simulink model "Feedback_linearization_3body_2body"  (R2019a)
settings: Solver=FixedStepAuto  StartTime=0.0  StopTime=5  FixedStep=0.001  RelTol=1e-7
libraries: simulink x1
settings Model: Creator=tommaso  LastModifiedBy=tommaso

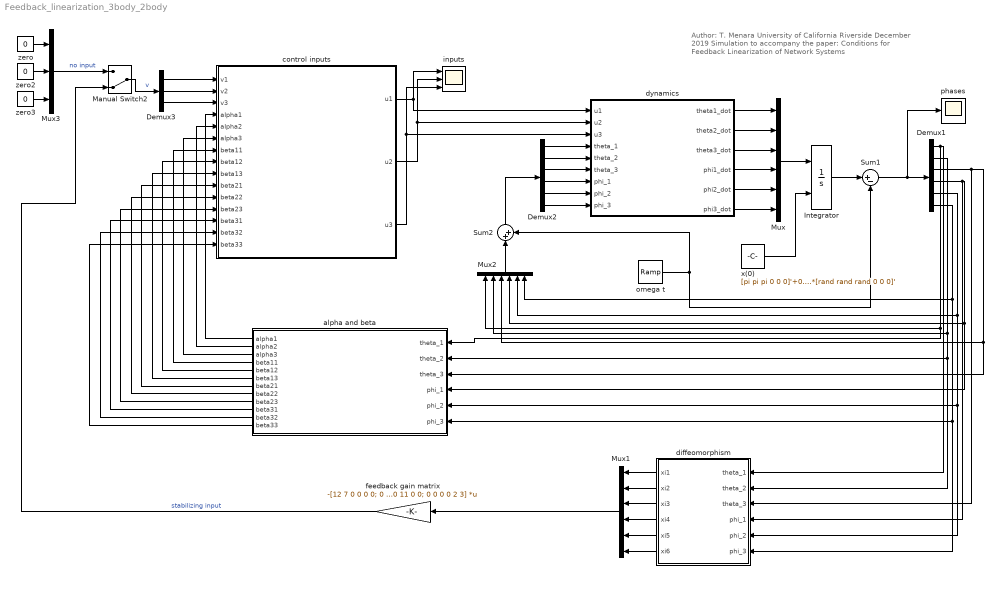
== system Feedback_linearization_3body_2body ==
  note: Author: T. Menara
      | University of California Riverside
      | December 2019
      |
      | Simulation to accompany the paper:
      | Conditions for Feedback Linearization of Network Systems
  Demux1 : Demux  Outputs=6
  Demux2 : Demux  Outputs=6
  Demux3 : Demux  Outputs=3
  Integrator : Integrator  InitialConditionSource=external  ContinuousStateAttributes='phases'
  Manual Switch2 : ManualSwitch  CurrentSetting=0
  Mux : Mux  Inputs=6
  Mux1 : Mux  Inputs=6
  Mux2 : Mux  Inputs=6
  Mux3 : Mux  Inputs=3
  Sum1 : Sum  Inputs=|+-
  Sum2 : Sum  Inputs=|++
  alpha and beta : Subsystem
  control inputs : Subsystem
  diffeomorphism : MATLAB Function  TreatAsAtomicUnit=on
  dynamics : MATLAB Function  TreatAsAtomicUnit=on
  feedback gain matrix : Gain  Gain=-[12 7 0 0 0 0; 0 0 30 11 0 0; 0 0 0 0 2 3]  Multiplication=Matrix(K*u) (u vector)
  inputs : Scope  NumInputPorts=3
  omega t : simulink/Sources/Ramp  slope=1  start=0  InitialOutput=0
  phases : Scope
  x(0) : Constant  Value=[pi pi pi 0 0 0]'+0.1*rand(6,1)-0.1*[rand rand rand 0 0 0]'
  zero : Constant  Value=0
  zero2 : Constant  Value=0
  zero3 : Constant  Value=0
  wires:
  dynamics/1(theta1_dot) -> Mux/1
  dynamics/2(theta2_dot) -> Mux/2
  Mux/1 -> Integrator/1
  feedback gain matrix/1 -> Manual Switch2/2  "stabilizing input"
  x(0)/1 -> Integrator/2
  dynamics/3(theta3_dot) -> Mux/3
  Demux1/1 -> Mux2/1, alpha and beta/1(theta_1), diffeomorphism/1(theta_1)
  Demux1/2 -> alpha and beta/2(theta_2), diffeomorphism/2(theta_2), Mux2/2
  Demux1/3 -> alpha and beta/3(theta_3), Mux2/3, diffeomorphism/3(theta_3)
  Manual Switch2/1 -> Demux3/1  "v"
  zero/1 -> Mux3/1
  diffeomorphism/1(xi1) -> Mux1/1
  diffeomorphism/2(xi2) -> Mux1/2
  diffeomorphism/3(xi3) -> Mux1/3
  Mux1/1 -> feedback gain matrix/1
  Sum1/1 -> Demux1/1, phases/1
  Integrator/1 -> Sum1/1
  Sum2/1 -> Demux2/1
  Mux2/1 -> Sum2/1
  omega t/1 -> Sum1/2, Sum2/2
  Demux2/1 -> dynamics/4(theta_1)
  Demux2/2 -> dynamics/5(theta_2)
  Demux2/3 -> dynamics/6(theta_3)
  dynamics/4(phi1_dot) -> Mux/4
  dynamics/5(phi2_dot) -> Mux/5
  dynamics/6(phi3_dot) -> Mux/6
  Demux2/4 -> dynamics/7(phi_1)
  Demux2/5 -> dynamics/8(phi_2)
  Demux2/6 -> dynamics/9(phi_3)
  Demux1/4 -> alpha and beta/4(phi_1), Mux2/4, diffeomorphism/4(phi_1)
  Demux1/5 -> diffeomorphism/5(phi_2), alpha and beta/5(phi_2), Mux2/5
  Demux1/6 -> alpha and beta/6(phi_3), diffeomorphism/6(phi_3), Mux2/6
  diffeomorphism/4(xi4) -> Mux1/4
  diffeomorphism/5(xi5) -> Mux1/5
  diffeomorphism/6(xi6) -> Mux1/6
  zero2/1 -> Mux3/2
  zero3/1 -> Mux3/3
  Mux3/1 -> Manual Switch2/1  "no input"
  control inputs/2(u2) -> inputs/2, dynamics/2(u2)
  control inputs/3(u3) -> inputs/3, dynamics/3(u3)
  control inputs/1(u1) -> inputs/1, dynamics/1(u1)
  Demux3/1 -> control inputs/1(v1)
  Demux3/2 -> control inputs/2(v2)
  Demux3/3 -> control inputs/3(v3)
  alpha and beta/1(alpha1) -> control inputs/4(alpha1)
  alpha and beta/2(alpha2) -> control inputs/5(alpha2)
  alpha and beta/3(alpha3) -> control inputs/6(alpha3)
  alpha and beta/4(beta11) -> control inputs/7(beta11)
  alpha and beta/5(beta12) -> control inputs/8(beta12)
  alpha and beta/6(beta13) -> control inputs/9(beta13)
  alpha and beta/7(beta21) -> control inputs/10(beta21)
  alpha and beta/8(beta22) -> control inputs/11(beta22)
  alpha and beta/9(beta23) -> control inputs/12(beta23)
  alpha and beta/10(beta31) -> control inputs/13(beta31)
  alpha and beta/11(beta32) -> control inputs/14(beta32)
  alpha and beta/12(beta33) -> control inputs/15(beta33)

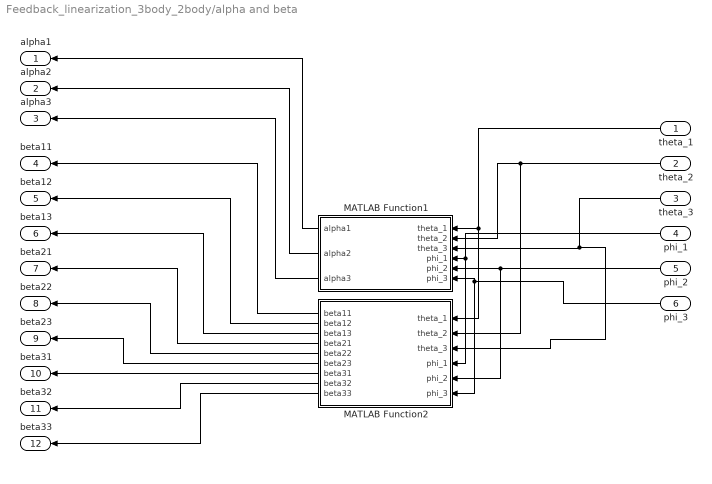
== system Feedback_linearization_3body_2body/alpha and beta ==
  theta_1 : Inport
  theta_2 : Inport  Port=2
  theta_3 : Inport  Port=3
  phi_1 : Inport  Port=4
  phi_2 : Inport  Port=5
  phi_3 : Inport  Port=6
  MATLAB Function1 : MATLAB Function  TreatAsAtomicUnit=on
  MATLAB Function2 : MATLAB Function  TreatAsAtomicUnit=on
  alpha1 : Outport
  alpha2 : Outport  Port=2
  alpha3 : Outport  Port=3
  beta11 : Outport  Port=4
  beta12 : Outport  Port=5
  beta13 : Outport  Port=6
  beta21 : Outport  Port=7
  beta22 : Outport  Port=8
  beta23 : Outport  Port=9
  beta31 : Outport  Port=10
  beta32 : Outport  Port=11
  beta33 : Outport  Port=12
  wires:
  MATLAB Function2/9(beta33) -> beta33/1
  MATLAB Function2/6(beta23) -> beta23/1
  theta_3/1 -> MATLAB Function2/3(theta_3), MATLAB Function1/3(theta_3)
  MATLAB Function1/2(alpha2) -> alpha2/1
  MATLAB Function1/3(alpha3) -> alpha3/1
  MATLAB Function2/1(beta11) -> beta11/1
  MATLAB Function2/7(beta31) -> beta31/1
  MATLAB Function2/5(beta22) -> beta22/1
  phi_1/1 -> MATLAB Function2/4(phi_1), MATLAB Function1/4(phi_1)
  MATLAB Function2/8(beta32) -> beta32/1
  phi_3/1 -> MATLAB Function1/6(phi_3), MATLAB Function2/6(phi_3)
  theta_1/1 -> MATLAB Function2/1(theta_1), MATLAB Function1/1(theta_1)
  MATLAB Function2/4(beta21) -> beta21/1
  MATLAB Function2/3(beta13) -> beta13/1
  theta_2/1 -> MATLAB Function2/2(theta_2), MATLAB Function1/2(theta_2)
  MATLAB Function1/1(alpha1) -> alpha1/1
  MATLAB Function2/2(beta12) -> beta12/1
  phi_2/1 -> MATLAB Function2/5(phi_2), MATLAB Function1/5(phi_2)

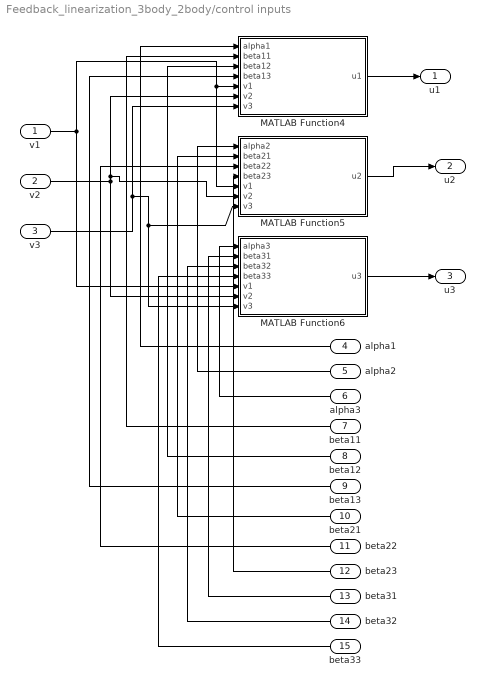
== system Feedback_linearization_3body_2body/control inputs ==
  v1 : Inport
  v2 : Inport  Port=2
  v3 : Inport  Port=3
  alpha1 : Inport  Port=4
  alpha2 : Inport  Port=5
  alpha3 : Inport  Port=6
  beta11 : Inport  Port=7
  beta12 : Inport  Port=8
  beta13 : Inport  Port=9
  beta21 : Inport  Port=10
  beta22 : Inport  Port=11
  beta23 : Inport  Port=12
  beta31 : Inport  Port=13
  beta32 : Inport  Port=14
  beta33 : Inport  Port=15
  MATLAB Function4 : MATLAB Function  TreatAsAtomicUnit=on
  MATLAB Function5 : MATLAB Function  TreatAsAtomicUnit=on
  MATLAB Function6 : MATLAB Function  TreatAsAtomicUnit=on
  u1 : Outport
  u2 : Outport  Port=2
  u3 : Outport  Port=3
  wires:
  beta13/1 -> MATLAB Function4/4(beta13)
  alpha3/1 -> MATLAB Function6/1(alpha3)
  beta23/1 -> MATLAB Function5/4(beta23)
  alpha2/1 -> MATLAB Function5/1(alpha2)
  beta32/1 -> MATLAB Function6/3(beta32)
  beta22/1 -> MATLAB Function5/3(beta22)
  beta12/1 -> MATLAB Function4/3(beta12)
  beta33/1 -> MATLAB Function6/4(beta33)
  beta31/1 -> MATLAB Function6/2(beta31)
  MATLAB Function5/1(u2) -> u2/1
  beta21/1 -> MATLAB Function5/2(beta21)
  alpha1/1 -> MATLAB Function4/1(alpha1)
  beta11/1 -> MATLAB Function4/2(beta11)
  v1/1 -> MATLAB Function6/5(v1), MATLAB Function4/5(v1), MATLAB Function5/5(v1)
  MATLAB Function4/1(u1) -> u1/1
  MATLAB Function6/1(u3) -> u3/1
  v3/1 -> MATLAB Function6/7(v3), MATLAB Function5/7(v3), MATLAB Function4/7(v3)
  v2/1 -> MATLAB Function5/6(v2), MATLAB Function4/6(v2), MATLAB Function6/6(v2)

== matlab function Feedback_linearization_3body_2body/alpha and beta/MATLAB Function1 ==
  data: alpha1 output; theta_1 input; theta_2 input; theta_3 input; phi_1 input; phi_2 input; phi_3 input; alpha2 output; alpha3 output
function [alpha1, alpha2, alpha3] = alpha_x(theta_1, theta_2, theta_3, phi_1, phi_2, phi_3)

d = 1;
k1 = 1;
k2 = 1;
N = 3;
omega = 0;

f =[omega + k1/N^2 * sin(theta_3 + theta_2 -2*theta_1); ...
 omega + k1/N^2 * sin(theta_3 + theta_1 -2*theta_2);...
 omega + k1/N^2 * sin(theta_1 + theta_2 -2*theta_3);...
 omega + k2/N * (sin(phi_2-phi_1) + sin(phi_3-phi_1)) + d*sin(theta_1-phi_1);...
 omega + k2/N * (sin(phi_1-phi_2) + sin(phi_3-phi_2)) + d*sin(theta_2-phi_2);...
 omega + k2/N * (sin(phi_1-phi_3) + sin(phi_2-phi_3)) + d*sin(theta_3-phi_3)];

J = [ -(2*k1*cos(theta_2 - 2*theta_1 + theta_3))/N^2,    (k1*cos(theta_2 - 2*theta_1 + theta_3))/N^2,    (k1*cos(theta_2 - 2*theta_1 + theta_3))/N^2,                                                                           0,                                                                           0,                                                                           0;...
    (k1*cos(theta_1 - 2*theta_2 + theta_3))/N^2, -(2*k1*cos(theta_1 - 2*theta_2 + theta_3))/N^2,    (k1*cos(theta_1 - 2*theta_2 + theta_3))/N^2,                                                                           0,                                                                           0,                                                                           0;...
    (k1*cos(theta_1 + theta_2 - 2*theta_3))/N^2,    (k1*cos(theta_1 + theta_2 - 2*theta_3))/N^2, -(2*k1*cos(theta_1 + theta_2 - 2*theta_3))/N^2,                                                                           0,                                                                           0,                                                                           0;...
                         d*cos(phi_1 - theta_1),                                              0,                                              0, - d*cos(phi_1 - theta_1) - (k2*(cos(phi_1 - phi_2) + cos(phi_1 - phi_3)))/N,                                                   (k2*cos(phi_1 - phi_2))/N,                                                   (k2*cos(phi_1 - phi_3))/N;...
                                              0,                         d*cos(phi_2 - theta_2),                                              0,                                                   (k2*cos(phi_1 - phi_2))/N, - d*cos(phi_2 - theta_2) - (k2*(cos(phi_1 - phi_2) + cos(phi_2 - phi_3)))/N,                                                   (k2*cos(phi_2 - phi_3))/N;...
                                              0,                                              0,                         d*cos(phi_3 - theta_3),                                                   (k2*cos(phi_1 - phi_3))/N,                                                   (k2*cos(phi_2 - phi_3))/N, - d*cos(phi_3 - theta_3) - (k2*(cos(phi_1 - phi_3) + cos(phi_2 - phi_3)))/N];

A = [J(4,1) J(4,2) J(4,3); J(5,1) J(5,2) J(5,3); J(6,1) J(6,2) J(6,3)];

% b = [(d*cos(phi_1 - theta_1) + (k2*(cos(phi_1 - phi_2) + cos(phi_1 - phi_3)))/N)*(d*sin(phi_1 - theta_1) - omega + (k2*(sin(phi_1 - phi_2) + sin(phi_1 - phi_3)))/N) + d*cos(phi_1 - theta_1)*(omega + (k1*sin(theta_2 - 2*theta_1 + theta_3))/N^2) + (k2*cos(phi_1 - phi_3)*(omega - d*sin(phi_3 - theta_3) + (k2*(sin(phi_1 - phi_3) + sin(phi_2 - phi_3)))/N))/N + (k2*cos(phi_1 - phi_2)*(omega - d*sin(phi_2 - theta_2) + (k2*(sin(phi_1 - phi_2) - sin(phi_2 - phi_3)))/N))/N;...
%  d*cos(phi_2 - theta_2)*(omega + (k1*sin(theta_1 - 2*theta_2 + theta_3))/N^2) - (d*cos(phi_2 - theta_2) + (k2*(cos(phi_1 - phi_2) + cos(phi_2 - phi_3)))/N)*(omega - d*sin(phi_2 - theta_2) + (k2*(sin(phi_1 - phi_2) - sin(phi_2 - phi_3)))/N) + (k2*cos(phi_2 - phi_3)*(omega - d*sin(phi_3 - theta_3) + (k2*(sin(phi_1 - phi_3) + sin(phi_2 - phi_3)))/N))/N - (k2*cos(phi_1 - phi_2)*(d*sin(phi_1 - theta_1) - omega + (k2*(sin(phi_1 - phi_2) + sin(phi_1 - phi_3)))/N))/N;...
%  d*cos(phi_3 - theta_3)*(omega + (k1*sin(theta_1 + theta_2 - 2*theta_3))/N^2) - (d*cos(phi_3 - theta_3) + (k2*(cos(phi_1 - phi_3) + cos(phi_2 - phi_3)))/N)*(omega - d*sin(phi_3 - theta_3) + (k2*(sin(phi_1 - phi_3) + sin(phi_2 - phi_3)))/N) - (k2*cos(phi_1 - phi_3)*(d*sin(phi_1 - theta_1) - omega + (k2*(sin(phi_1 - phi_2) + sin(phi_1 - phi_3)))/N))/N + (k2*cos(phi_2 - phi_3)*(omega - d*sin(phi_2 - theta_2) + (k2*(sin(phi_1 - phi_2) - sin(phi_2 - phi_3)))/N))/N];

b = [J(4,:)*f; J(5,:)*f; J(6,:)*f];

temp = -inv(A)*b;

alpha1 = temp(1);
alpha2 = temp(2);
alpha3 = temp(3);

== matlab function Feedback_linearization_3body_2body/dynamics ==
  data: u1 input; u2 input; u3 input; theta1_dot output; theta_1 input; theta_2 input; theta2_dot output; theta_3 input; theta3_dot output; phi_1 input; phi_2 input; phi_3 input; phi1_dot output; phi2_dot output; phi3_dot output
function [theta1_dot, theta2_dot, theta3_dot, phi1_dot, phi2_dot, phi3_dot] = dynamics(u1, u2, u3, theta_1, theta_2, theta_3, phi_1, phi_2, phi_3)

d = 1;
k1 = 1;
k2 = 1;
N = 3;
omega = 1;

theta1_dot = omega + k1/N^2 * sin(theta_3 + theta_2 -2*theta_1) + u1;
theta2_dot = omega + k1/N^2 * sin(theta_3 + theta_1 -2*theta_2) + u2;
theta3_dot = omega + k1/N^2 * sin(theta_1 + theta_2 -2*theta_3) + u3;
phi1_dot =  omega + k2/N * (sin(phi_2-phi_1) + sin(phi_3-phi_1)) + d*sin(theta_1-phi_1);
phi2_dot = omega + k2/N * (sin(phi_1-phi_2) + sin(phi_3-phi_2)) + d*sin(theta_2-phi_2);
phi3_dot = omega + k2/N * (sin(phi_1-phi_3) + sin(phi_2-phi_3)) + d*sin(theta_3-phi_3);

== matlab function Feedback_linearization_3body_2body/alpha and beta/MATLAB Function2 ==
  data: beta11 output; theta_1 input; theta_2 input; theta_3 input; phi_1 input; phi_2 input; phi_3 input; beta12 output; beta13 output; beta21 output; beta22 output; beta23 output; beta31 output; beta32 output; beta33 output
function [beta11, beta12, beta13, beta21, beta22, beta23, beta31, beta32, beta33] = beta_x(theta_1, theta_2, theta_3, phi_1, phi_2, phi_3)

d = 1;
k1 = 1;
k2 = 1;
N = 3;
omega = 0;

% J = [ -(2*k1*cos(theta_2 - 2*theta_1 + theta_3))/N^2,    (k1*cos(theta_2 - 2*theta_1 + theta_3))/N^2,    (k1*cos(theta_2 - 2*theta_1 + theta_3))/N^2,                                                                           0,                                                                           0,                                                                           0;...
%     (k1*cos(theta_1 - 2*theta_2 + theta_3))/N^2, -(2*k1*cos(theta_1 - 2*theta_2 + theta_3))/N^2,    (k1*cos(theta_1 - 2*theta_2 + theta_3))/N^2,                                                                           0,                                                                           0,                                                                           0;...
%     (k1*cos(theta_1 + theta_2 - 2*theta_3))/N^2,    (k1*cos(theta_1 + theta_2 - 2*theta_3))/N^2, -(2*k1*cos(theta_1 + theta_2 - 2*theta_3))/N^2,                                                                           0,                                                                           0,                                                                           0;...
%                          d*cos(phi_1 - theta_1),                                              0,                                              0, - d*cos(phi_1 - theta_1) - (k2*(cos(phi_1 - phi_2) + cos(phi_1 - phi_3)))/N,                                                   (k2*cos(phi_1 - phi_2))/N,                                                   (k2*cos(phi_1 - phi_3))/N;...
%                                               0,                         d*cos(phi_2 - theta_2),                                              0,                                                   (k2*cos(phi_1 - phi_2))/N, - d*cos(phi_2 - theta_2) - (k2*(cos(phi_1 - phi_2) + cos(phi_2 - phi_3)))/N,                                                   (k2*cos(phi_2 - phi_3))/N;...
%                                               0,                                              0,                         d*cos(phi_3 - theta_3),                                                   (k2*cos(phi_1 - phi_3))/N,                                                   (k2*cos(phi_2 - phi_3))/N, - d*cos(phi_3 - theta_3) - (k2*(cos(phi_1 - phi_3) + cos(phi_2 - phi_3)))/N];

% A = [J(4,1) J(4,2) J(4,3); J(5,1) J(5,2) J(5,3); J(6,1) J(6,2) J(6,3)];

% temp = inv(A);

% beta11 = temp(1,1);
% beta12 = temp(1,2);
% beta13 = temp(1,3);
% beta21 = temp(2,1);
% beta22 = temp(2,2);
% beta23 = temp(2,3);
% beta31 = temp(3,1);
% beta32 = temp(3,2);
% beta33 = temp(3,3);


% they are actually easy to compute because A is diagonal:

beta11 = 1/(d*cos(phi_1 - theta_1));
beta12 = 0;
beta13 = 0;
beta21 = 0;
beta22 = 1/(d*cos(phi_2 - theta_2));
beta23 = 0;
beta31 = 0;
beta32 = 0;
beta33 = 1/(d*cos(phi_3 - theta_3));

== matlab function Feedback_linearization_3body_2body/diffeomorphism ==
  data: xi1 output; theta_1 input; theta_2 input; theta_3 input; xi2 output; xi3 output; phi_1 input; phi_2 input; phi_3 input; xi4 output; xi5 output; xi6 output
function [xi1, xi2, xi3, xi4, xi5, xi6] = phi(theta_1, theta_2, theta_3, phi_1, phi_2, phi_3)

d = 1;
k1 = 1;
k2 = 1;
N = 3;
omega = 0; % zero because of rotating frame

f =[omega + k1/N^2 * sin(theta_3 + theta_2 -2*theta_1); ...
 omega + k1/N^2 * sin(theta_3 + theta_1 -2*theta_2);...
 omega + k1/N^2 * sin(theta_1 + theta_2 -2*theta_3);...
 omega + k2/N * (sin(phi_2-phi_1) + sin(phi_3-phi_1)) + d*sin(theta_1-phi_1);...
 omega + k2/N * (sin(phi_1-phi_2) + sin(phi_3-phi_2)) + d*sin(theta_2-phi_2);...
 omega + k2/N * (sin(phi_1-phi_3) + sin(phi_2-phi_3)) + d*sin(theta_3-phi_3)];

J = [ -(2*k1*cos(theta_2 - 2*theta_1 + theta_3))/N^2,    (k1*cos(theta_2 - 2*theta_1 + theta_3))/N^2,    (k1*cos(theta_2 - 2*theta_1 + theta_3))/N^2,                                                                           0,                                                                           0,                                                                           0;...
    (k1*cos(theta_1 - 2*theta_2 + theta_3))/N^2, -(2*k1*cos(theta_1 - 2*theta_2 + theta_3))/N^2,    (k1*cos(theta_1 - 2*theta_2 + theta_3))/N^2,                                                                           0,                                                                           0,                                                                           0;...
    (k1*cos(theta_1 + theta_2 - 2*theta_3))/N^2,    (k1*cos(theta_1 + theta_2 - 2*theta_3))/N^2, -(2*k1*cos(theta_1 + theta_2 - 2*theta_3))/N^2,                                                                           0,                                                                           0,                                                                           0;...
                         d*cos(phi_1 - theta_1),                                              0,                                              0, - d*cos(phi_1 - theta_1) - (k2*(cos(phi_1 - phi_2) + cos(phi_1 - phi_3)))/N,                                                   (k2*cos(phi_1 - phi_2))/N,                                                   (k2*cos(phi_1 - phi_3))/N;...
                                              0,                         d*cos(phi_2 - theta_2),                                              0,                                                   (k2*cos(phi_1 - phi_2))/N, - d*cos(phi_2 - theta_2) - (k2*(cos(phi_1 - phi_2) + cos(phi_2 - phi_3)))/N,                                                   (k2*cos(phi_2 - phi_3))/N;...
                                              0,                                              0,                         d*cos(phi_3 - theta_3),                                                   (k2*cos(phi_1 - phi_3))/N,                                                   (k2*cos(phi_2 - phi_3))/N, - d*cos(phi_3 - theta_3) - (k2*(cos(phi_1 - phi_3) + cos(phi_2 - phi_3)))/N];


xi1 = phi_1;
xi2 = f(4,1);
xi3 = phi_2;
xi4 = f(5,1);
xi5 = phi_3;
xi6 = f(6,1);

== matlab function Feedback_linearization_3body_2body/control inputs/MATLAB Function4 ==
  data: u1 output; alpha1 input; beta11 input; beta12 input; beta13 input; v1 input; v2 input; v3 input
function u1  = control1(alpha1, beta11, beta12, beta13, v1, v2, v3)

u1 = alpha1 + beta11*v1;

== matlab function Feedback_linearization_3body_2body/control inputs/MATLAB Function5 ==
  data: u2 output; alpha2 input; beta21 input; beta22 input; beta23 input; v1 input; v2 input; v3 input
function u2  = control2(alpha2, beta21, beta22, beta23, v1, v2, v3)

u2 = alpha2 + beta22*v2;

== matlab function Feedback_linearization_3body_2body/control inputs/MATLAB Function6 ==
  data: u3 output; alpha3 input; beta31 input; beta32 input; beta33 input; v1 input; v2 input; v3 input
function u3  = control3(alpha3, beta31, beta32, beta33, v1, v2, v3)

u3 = alpha3 + beta33*v3;
